simulink model "System_02"  (R2020b)
settings: Solver=VariableStepAuto  StartTime=0.0  StopTime=15*3600  RelTol=1e-3
undefined symbols (not defined in the file or in its folder): J, Kd, Kf, Kg, Kt, L, R
libraries: pid_lib x1
settings Model: Creator=riwakaram  LastModifiedBy=riwakaram
settings DataIOCC: ExternalInput=[sunTime, sunPosition]  LoadExternalInput=on

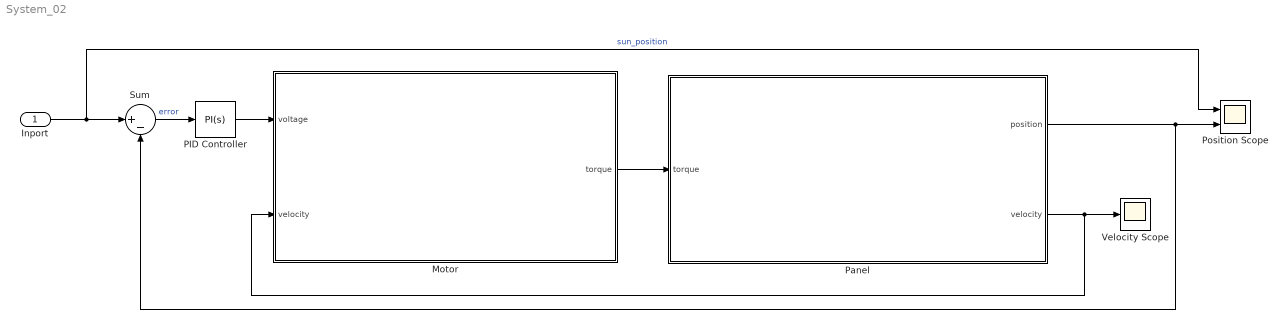
== system System_02 ==
  Inport : Inport
  Motor : Subsystem
  PID Controller : pid_lib/PID Controller  Controller=PI  Form=Parallel  TimeDomain=Continuous-time  UseExternalTs=off  SampleTime=-1  IntegratorMethod=Forward Euler  FilterMethod=Forward Euler  ControllerParametersSource=internal  P=240  I=180  D=0  UseFilter=on  N=100  TunerSelectOption=Transfer Function Based (PID Tuner App)  InitialConditionSource=internal  InitialConditionForIntegrator=0  InitialConditionForFilter=0  DifferentiatorICPrevScaledInput=0  ExternalReset=none  TrackingMode=off  Kt=1  LimitOutput=off  SatLimitsSource=internal  UpperSaturationLimit=inf  LowerSaturationLimit=-inf  LinearizeAsGain=on  AntiWindupMode=none  Kb=1  POutMin=[]  POutMax=[]  IOutMin=[]  IOutMax=[]  DOutMin=[]  DOutMax=[]  NOutMin=[]  NOutMax=[]  SumOutMin=[]  SumOutMax=[]  SaturationOutMin=[]  SaturationOutMax=[]  PParamMin=[]  PParamMax=[]  IParamMin=[]  IParamMax=[]  DParamMin=[]  DParamMax=[]  NParamMin=[]  NParamMax=[]  KbParamMin=[]  KbParamMax=[]  KtParamMin=[]  KtParamMax=[]  KbOutMin=[]  KbOutMax=[]  KtOutMin=[]  KtOutMax=[]  IntegratorOutMin=[]  IntegratorOutMax=[]  FilterOutMin=[]  FilterOutMax=[]  SumI1OutMin=[]  SumI1OutMax=[]  SumI2OutMin=[]  SumI2OutMax=[]  SumI3OutMin=[]  SumI3OutMax=[]  SumI4OutMin=[]  SumI4OutMax=[]  SumDOutMin=[]  SumDOutMax=[]  DifferentiatorOutMin=[]  DifferentiatorOutMax=[]  FilterDiffOutCoefMin=[]  FilterDiffOutCoefMax=[]  ReciprocalOutMin=[]  ReciprocalOutMax=[]  SumDenOutMin=[]  SumDenOutMax=[]  SumNumOutMin=[]  SumNumOutMax=[]  DivideOutMin=[]  DivideOutMax=[]  UdiffTsProdOutMin=[]  UdiffTsProdOutMax=[]  NTsProdOutMin=[]  NTsProdOutMax=[]  UintegralTsProdOutMin=[]  UintegralTsProdOutMax=[]  UngainTsProdOutMin=[]  UngainTsProdOutMax=[]  IntegratorContinuousStateAttributes=''  IntegratorStateMustResolveToSignalObject=off  IntegratorRTWStateStorageClass=Auto  FilterContinuousStateAttributes=''  FilterStateMustResolveToSignalObject=off  FilterRTWStateStorageClass=Auto  ParallelPVariant=InternalParameters  IdealPVariant=Disabled  IVariant=InternalParameters  DVariant=Disabled  IntegratorVariant=Continuous  SatVariant=Disabled  AWVariant=Passthrough  PCopyVariant=Disabled  TRVariant=Disabled  FdbkBlocksVariant=Forward  IdealPFdbkVariant=Disabled  SatFdbkVariant=Disabled  DerivativeFilterVariant=Disabled  NVariant=Disabled  NCopyVariant=Disabled_SignalSpec  FilterICVariant=Disabled  IntegratorICVariant=InternalICs  ExternalResetVariant=Disabled  TRSumVariant=Passthrough  SumFdbkVariant=Disabled  SumVariant=Sum_PI  TsampFilterVariant=InternalTs  TsampNgainVariant=Passthrough  TsampIntegralVariant=Passthrough  ExternalSaturationOutDataTypeStr=Inherit: Same as second input
  Panel : Subsystem
  Position Scope : Scope  NumInputPorts=2
  Sum : Sum  Inputs=|+-
  Velocity Scope : Scope
  wires:
  Panel/2(velocity) -> Velocity Scope/1, Motor/2(velocity)
  PID Controller/1 -> Motor/1(voltage)
  Sum/1 -> PID Controller/1  "error"
  Inport/1 -> Position Scope/1, Sum/1  "sun_position"
  Motor/1(torque) -> Panel/1(torque)
  Panel/1(position) -> Sum/2, Position Scope/2

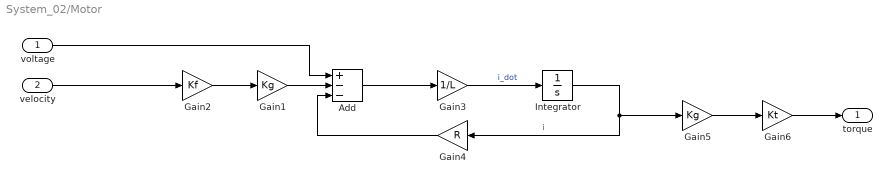
== system System_02/Motor ==
  voltage : Inport
  velocity : Inport  Port=2
  Add : Sum  Inputs=+--
  Gain1 : Gain  Gain=Kg
  Gain2 : Gain  Gain=Kf
  Gain3 : Gain  Gain=1/L
  Gain4 : Gain  Gain=R
  Gain5 : Gain  Gain=Kg
  Gain6 : Gain  Gain=Kt
  Integrator : Integrator
  torque : Outport
  wires:
  Gain1/1 -> Add/2
  voltage/1 -> Add/1
  Gain4/1 -> Add/3
  velocity/1 -> Gain2/1
  Gain2/1 -> Gain1/1
  Integrator/1 -> Gain5/1, Gain4/1  "i"
  Add/1 -> Gain3/1
  Gain3/1 -> Integrator/1  "i_dot"
  Gain5/1 -> Gain6/1
  Gain6/1 -> torque/1

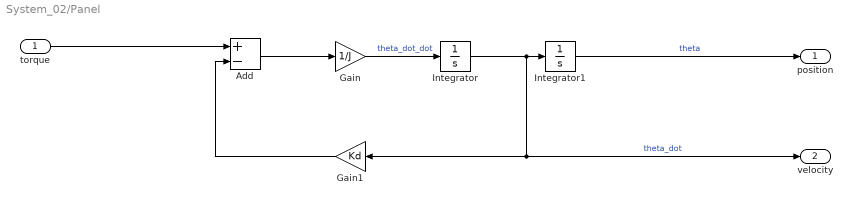
== system System_02/Panel ==
  torque : Inport
  Add : Sum  Inputs=+-
  Gain : Gain  Gain=1/J
  Gain1 : Gain  Gain=Kd
  Integrator : Integrator
  Integrator1 : Integrator
  position : Outport
  velocity : Outport  Port=2
  wires:
  torque/1 -> Add/1
  Gain1/1 -> Add/2
  Gain/1 -> Integrator/1  "theta_dot_dot"
  Add/1 -> Gain/1
  Integrator1/1 -> position/1  "theta"
  Integrator/1 -> Gain1/1, velocity/1, Integrator1/1  "theta_dot"
